simulink model "example4"  (R2017a)
settings: Solver=FixedStepAuto  StartTime=0.0  StopTime=10.0  RelTol=1e-3
settings Model: Creator=rober  LastModifiedBy=rober
settings SolverCC: AutoInsertRateTranBlk=on

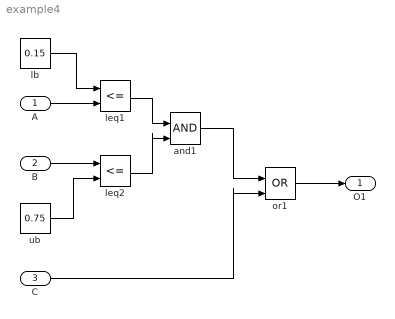
== system example4 ==
  A : Inport  OutDataTypeStr=single
  B : Inport  Port=2  OutDataTypeStr=single
  C : Inport  Port=3  OutDataTypeStr=boolean
  and1 : Logic  IconShape=distinctive  AllPortsSameDT=off  OutDataTypeStr=boolean
  lb : Constant  Value=0.15  OutDataTypeStr=single
  leq1 : RelationalOperator  Operator=<=  OutDataTypeStr=boolean  RndMeth=Simplest
  leq2 : RelationalOperator  Operator=<=  OutDataTypeStr=boolean  RndMeth=Simplest
  or1 : Logic  Operator=OR  IconShape=distinctive  AllPortsSameDT=off  OutDataTypeStr=boolean
  ub : Constant  Value=0.75  OutDataTypeStr=single
  O1 : Outport
  wires:
  and1/1 -> or1/1
  C/1 -> or1/2
  or1/1 -> O1/1
  lb/1 -> leq1/1
  A/1 -> leq1/2
  B/1 -> leq2/1
  ub/1 -> leq2/2
  leq2/1 -> and1/2
  leq1/1 -> and1/1
